simulink model "task43"  (R2015b)
settings: Solver=VariableStepAuto  StartTime=0.0  StopTime=10.0  RelTol=1e-3
settings Model: Creator=Martin  LastModifiedBy=Martin

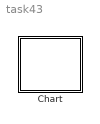
== system task43 ==
  Chart : Stateflow chart  TreatAsAtomicUnit=on

== stateflow chart task43/Chart ==
  state IEI
  state IEP
  state IED
  state IFI
  state IFP
  state IFD
  state PEI
  state PEP
  state PED
  state PFI
  state PFP
  state PFD
  state DEI
  state DEP
  state DED
  state DFI
  state DFP
  state DFD
  IFP -> IEP [order 2]
  PEI -> IFI [order 3]
  IFD -> IFI
  IED -> IEI
  IEP -> IED [order 2]
  IFP -> IFI [order 1]
  (default) -> IEI
  IFI -> IFP
  IEP -> IEI [order 1]
  DFD -> IFD [order 1]
  DEI -> IEI
  DFP -> IFP [order 3]
  DFI -> IFI
  PFI -> IFI [order 1]
  DEP -> IEP [order 1]
  IEI -> PEI
  IEP -> PEP [order 3]
  PFP -> IFP [order 3]
  PFD -> IFD [order 3]
  PED -> PFD [order 3]
  PFP -> PFD [order 2]
  PEI -> PFI [order 2]
  PEP -> PED [order 3]
  PEP -> PEI [order 4]
  PFD -> PFI [order 2]
  PED -> PEI [order 2]
  PFI -> PFP [order 3]
  PEP -> PFP [order 2]
  PFD -> DFD [order 1]
  PEI -> DEI [order 1]
  PEP -> DEP [order 1]
  PFP -> PEP [order 5]
  PED -> DED [order 1]
  PFI -> DFI [order 2]
  PFP -> PFI [order 4]
  PFP -> DFP [order 1]
  DEP -> DEI [order 2]
  DEP -> DED [order 3]
  DED -> DEI
  DFP -> DEP [order 4]
  DFD -> DFI [order 2]
  DFP -> DFI [order 1]
  DFP -> DFD [order 2]
